simulink model "ffffff"  (R2021b)
settings: Solver=VariableStepAuto  StartTime=0.0  StopTime=25  RelTol=1e-3
values from neighbouring files (symbols this model uses):
  Ad1 = Ad1 + ((A*Ts1)^i)/factorial(i)    [untitled2.m]
  Ad11 = Ad11 + ((A11*Ts)^i)/factorial(i)    [untitled2.m]
  Ad11_1 = Ad11_1 + ((A11*Ts1)^i)/factorial(i)    [untitled2.m]
  Ad11_2 = Ad11_2 + ((A11*Ts2)^i)/factorial(i)    [untitled2.m]
  Ad2 = Ad2 + ((A*Ts2)^i)/factorial(i)    [untitled2.m]
  Ad22 = Ad22 + ((A22*Ts)^i)/factorial(i)    [untitled2.m]
  Ad22_1 = Ad22_1 + ((A22*Ts1)^i)/factorial(i)    [untitled2.m]
  Ad22_2 = Ad22_2 + ((A22*Ts2)^i)/factorial(i)    [untitled2.m]
  Bd1 = inv(A)*(Ad1-I)*B    [untitled2.m]
  Bd11 = inv(A11)*(Ad11-I11)*B11    [untitled2.m]
  Bd11_1 = inv(A11)*(Ad11_1-I11)*B11    [untitled2.m]
  Bd11_2 = inv(A11)*(Ad11_2-I11)*B11    [untitled2.m]
  Bd2 = inv(A)*(Ad2-I)*B    [untitled2.m]
  Bd22 = [0;0]    [untitled2.m]
  Bd22_1 = [0;0]    [untitled2.m]
  Bd22_2 = [0;0]    [untitled2.m]
  C = [0 0 0.1]    [untitled2.m]
  C11 = [1]    [untitled2.m]
  C22 = [1 0]    [untitled2.m]
  Ts = 1/100    (= 0.01)    [untitled2.m]
  Ts1 = 1/10    (= 0.1)    [untitled2.m]
  Ts2 = 1/5    (= 0.2)    [untitled2.m]
settings Model: Creator=wen  LastModifiedBy=wen

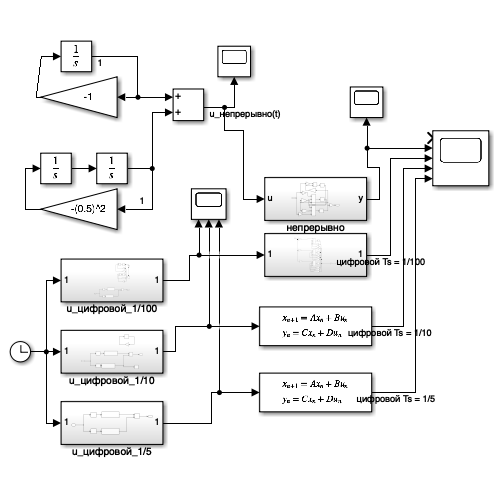
[thumbnail: Simulink's stored preview of the top-level diagram]
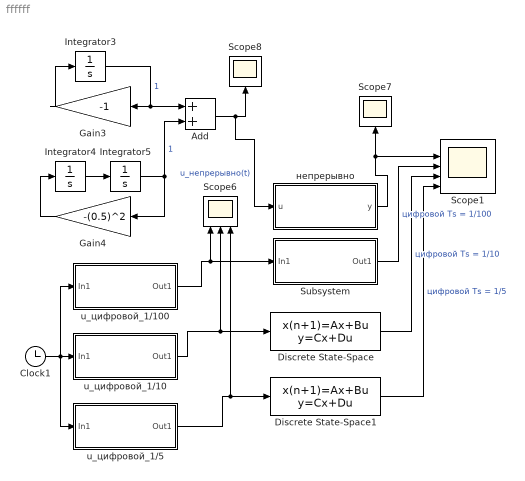
== system ffffff ==
  Add : Sum
  Clock1 : Clock
  Discrete State-Space : DiscreteStateSpace  A=Ad1  B=Bd1  C=C  D=0  SampleTime=Ts1
  Discrete State-Space1 : DiscreteStateSpace  A=Ad2  B=Bd2  C=C  D=0  SampleTime=Ts2
  Gain3 : Gain  Gain=-1
  Gain4 : Gain  Gain=-(0.5)^2
  Integrator3 : Integrator  InitialCondition=3
  Integrator4 : Integrator  InitialCondition=sqrt(2)/2*0.5*(-0.5)
  Integrator5 : Integrator  InitialCondition=0.5*sqrt(2)/2
  Scope1 : Scope  NumInputPorts=5
  Scope6 : Scope  NumInputPorts=3
  Scope7 : Scope
  Scope8 : Scope
  Subsystem : Subsystem
  u_цифровой_1/10 : Subsystem
  u_цифровой_1/100 : Subsystem
  u_цифровой_1/5 : Subsystem
  непрерывно : Subsystem
  wires:
  непрерывно/1(y) -> Scope7/1, Scope1/2
  Subsystem/1(Out1) -> Scope1/3  "цифровой Ts = 1/100"
  Discrete State-Space/1 -> Scope1/4  "цифровой Ts = 1/10"
  Discrete State-Space1/1 -> Scope1/5  "цифровой Ts = 1/5"
  u_цифровой_1/100/1(Out1) -> Subsystem/1(In1), Scope6/1
  u_цифровой_1/10/1(Out1) -> Discrete State-Space/1, Scope6/2
  u_цифровой_1/5/1(Out1) -> Discrete State-Space1/1, Scope6/3
  Clock1/1 -> u_цифровой_1/5/1(In1), u_цифровой_1/10/1(In1), u_цифровой_1/100/1(In1)
  Integrator3/1 -> Add/1, Gain3/1  "1"
  Gain3/1 -> Integrator3/1
  Gain4/1 -> Integrator4/1
  Integrator4/1 -> Integrator5/1
  Integrator5/1 -> Gain4/1, Add/2  "1"
  Add/1 -> непрерывно/1(u), Scope8/1  "u_непрерывно(t)"

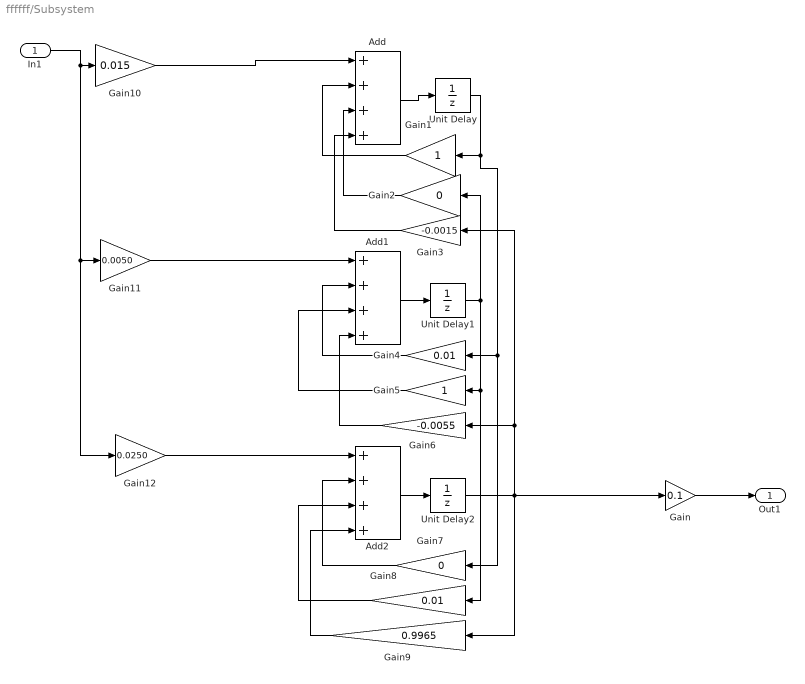
== system ffffff/Subsystem ==
  In1 : Inport
  Add : Sum  Inputs=++++
  Add1 : Sum  Inputs=++++
  Add2 : Sum  Inputs=++++
  Gain : Gain  Gain=0.1
  Gain1 : Gain
  Gain10 : Gain  Gain=0.015
  Gain11 : Gain  Gain=0.0050
  Gain12 : Gain  Gain=0.0250
  Gain2 : Gain  Gain=0
  Gain3 : Gain  Gain=-0.0015
  Gain4 : Gain  Gain=0.01
  Gain5 : Gain
  Gain6 : Gain  Gain=-0.0055
  Gain7 : Gain  Gain=0
  Gain8 : Gain  Gain=0.01
  Gain9 : Gain  Gain=0.9965
  Unit Delay : UnitDelay  SampleTime=Ts  HasFrameUpgradeWarning=on
  Unit Delay1 : UnitDelay  SampleTime=Ts  HasFrameUpgradeWarning=on
  Unit Delay2 : UnitDelay  SampleTime=Ts  HasFrameUpgradeWarning=on
  Out1 : Outport
  wires:
  Add/1 -> Unit Delay/1
  Add1/1 -> Unit Delay1/1
  Add2/1 -> Unit Delay2/1
  Gain/1 -> Out1/1
  Unit Delay2/1 -> Gain9/1, Gain3/1, Gain6/1, Gain/1
  In1/1 -> Gain12/1, Gain11/1, Gain10/1
  Gain10/1 -> Add/1
  Gain11/1 -> Add1/1
  Gain12/1 -> Add2/1
  Unit Delay/1 -> Gain7/1, Gain4/1, Gain1/1
  Unit Delay1/1 -> Gain2/1, Gain8/1, Gain5/1
  Gain1/1 -> Add/2
  Gain2/1 -> Add/3
  Gain3/1 -> Add/4
  Gain4/1 -> Add1/2
  Gain5/1 -> Add1/3
  Gain6/1 -> Add1/4
  Gain7/1 -> Add2/2
  Gain8/1 -> Add2/3
  Gain9/1 -> Add2/4

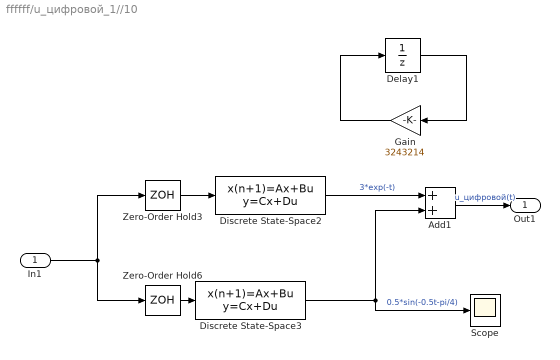
== system ffffff/u_цифровой_1//10 ==
  In1 : Inport
  Add1 : Sum
  Delay1 : UnitDelay  InitialCondition=0.3536  SampleTime=Ts  HasFrameUpgradeWarning=on
  Discrete State-Space2 : DiscreteStateSpace  A=Ad11_1  B=Bd11_1  C=C11  D=0  InitialCondition=3  SampleTime=Ts1
  Discrete State-Space3 : DiscreteStateSpace  A=Ad22_1  B=Bd22_1  C=C22  D=0  InitialCondition="[0.5*sqrt(2)/2  ; sqrt(2)/2*0.5*(-0.5)]"  SampleTime=Ts1
  Gain : Gain  Gain=3243214
  Scope : Scope
  Zero-Order Hold3 : ZeroOrderHold  SampleTime=Ts1
  Zero-Order Hold6 : ZeroOrderHold  SampleTime=Ts1
  Out1 : Outport
  wires:
  Add1/1 -> Out1/1  "u_цифровой(t)"
  Discrete State-Space2/1 -> Add1/1  "3*exp(-t)"
  Discrete State-Space3/1 -> Add1/2, Scope/1  "0.5*sin(-0.5t-pi/4)"
  Zero-Order Hold6/1 -> Discrete State-Space3/1
  Zero-Order Hold3/1 -> Discrete State-Space2/1
  In1/1 -> Zero-Order Hold6/1, Zero-Order Hold3/1
  Delay1/1 -> Gain/1
  Gain/1 -> Delay1/1

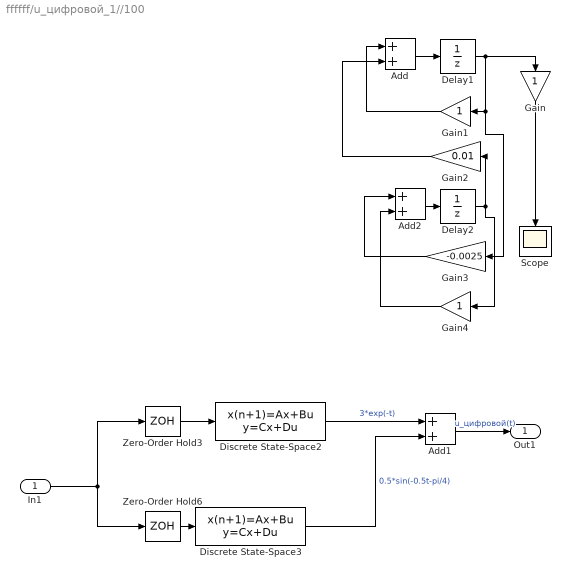
== system ffffff/u_цифровой_1//100 ==
  In1 : Inport
  " Delay2" : UnitDelay  InitialCondition=-0.1768  SampleTime=Ts  HasFrameUpgradeWarning=on
  Add : Sum
  Add1 : Sum
  Add2 : Sum
  Delay1 : UnitDelay  InitialCondition=0.3536  SampleTime=Ts  HasFrameUpgradeWarning=on
  Discrete State-Space2 : DiscreteStateSpace  A=Ad11  B=Bd11  C=C11  D=0  InitialCondition=3  SampleTime=Ts
  Discrete State-Space3 : DiscreteStateSpace  A=Ad22  B=Bd22  C=C22  D=0  InitialCondition="[0.5*sqrt(2)/2  ; sqrt(2)/2*0.5*(-0.5)]"  SampleTime=Ts
  Gain : Gain
  Gain1 : Gain
  Gain2 : Gain  Gain=0.01
  Gain3 : Gain  Gain=-0.0025
  Gain4 : Gain
  Scope : Scope
  Zero-Order Hold3 : ZeroOrderHold  SampleTime=Ts
  Zero-Order Hold6 : ZeroOrderHold  SampleTime=Ts
  Out1 : Outport
  wires:
  Add1/1 -> Out1/1  "u_цифровой(t)"
  Discrete State-Space2/1 -> Add1/1  "3*exp(-t)"
  Discrete State-Space3/1 -> Add1/2  "0.5*sin(-0.5t-pi/4)"
  Zero-Order Hold6/1 -> Discrete State-Space3/1
  Zero-Order Hold3/1 -> Discrete State-Space2/1
  In1/1 -> Zero-Order Hold6/1, Zero-Order Hold3/1
  Add/1 -> Delay1/1
  Add2/1 -> " Delay2"/1
  Gain1/1 -> Add/1
  " Delay2"/1 -> Gain4/1, Gain2/1
  Delay1/1 -> Gain/1, Gain3/1, Gain1/1
  Gain4/1 -> Add2/2
  Gain/1 -> Scope/1
  Gain2/1 -> Add/2
  Gain3/1 -> Add2/1

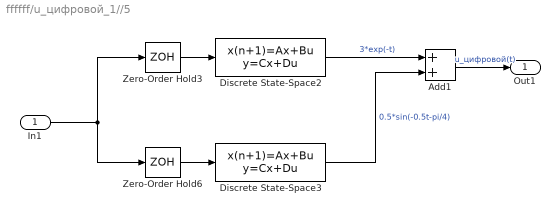
== system ffffff/u_цифровой_1//5 ==
  In1 : Inport
  Add1 : Sum
  Discrete State-Space2 : DiscreteStateSpace  A=Ad11_2  B=Bd11_2  C=C11  D=0  InitialCondition=3  SampleTime=Ts2
  Discrete State-Space3 : DiscreteStateSpace  A=Ad22_2  B=Bd22_2  C=C22  D=0  InitialCondition="[0.5*sqrt(2)/2  ; sqrt(2)/2*0.5*(-0.5)]"  SampleTime=Ts2
  Zero-Order Hold3 : ZeroOrderHold  SampleTime=Ts2
  Zero-Order Hold6 : ZeroOrderHold  SampleTime=Ts2
  Out1 : Outport
  wires:
  Add1/1 -> Out1/1  "u_цифровой(t)"
  Discrete State-Space2/1 -> Add1/1  "3*exp(-t)"
  Discrete State-Space3/1 -> Add1/2  "0.5*sin(-0.5t-pi/4)"
  Zero-Order Hold6/1 -> Discrete State-Space3/1
  Zero-Order Hold3/1 -> Discrete State-Space2/1
  In1/1 -> Zero-Order Hold6/1, Zero-Order Hold3/1

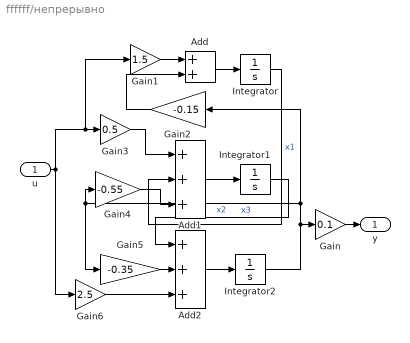
== system ffffff/непрерывно ==
  u : Inport
  Add : Sum
  Add1 : Sum  Inputs=+++
  Add2 : Sum  Inputs=+++
  Gain : Gain  Gain=0.1
  Gain1 : Gain  Gain=1.5
  Gain2 : Gain  Gain=-0.15
  Gain3 : Gain  Gain=0.5
  Gain4 : Gain  Gain=-0.55
  Gain5 : Gain  Gain=-0.35
  Gain6 : Gain  Gain=2.5
  Integrator : Integrator
  Integrator1 : Integrator
  Integrator2 : Integrator
  y : Outport
  wires:
  Integrator2/1 -> Gain/1, Gain4/1, Gain5/1, Gain2/1  "x3"
  Gain/1 -> y/1
  Integrator1/1 -> Add2/1  "x2"
  Integrator/1 -> Add1/2  "x1"
  Add/1 -> Integrator/1
  Gain2/1 -> Add/2
  Gain1/1 -> Add/1
  u/1 -> Gain1/1, Gain3/1, Gain6/1
  Add1/1 -> Integrator1/1
  Gain3/1 -> Add1/1
  Gain4/1 -> Add1/3
  Add2/1 -> Integrator2/1
  Gain5/1 -> Add2/2
  Gain6/1 -> Add2/3
